simulink library "ForcesHypothese"  (R2018a)
settings: Solver=VariableStepAuto  StartTime=0.0  StopTime=10.0  RelTol=1e-3
values from neighbouring files (symbols this model uses):
  w_alpha = 0    [LimitationVitesse.m]
  w_dist = 0    [LimitationVitesse.m]
settings Model: Creator=thomas.moser  LastModifiedBy=thomas.moser

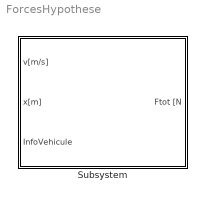
== system ForcesHypothese ==
  Subsystem : Subsystem  mask{rho=1.225, g=9.81}
      mask prompts: rho "Densité de l'air [kg/m^3] :"; g "Accélération gravitationelle [m/s^2] :"

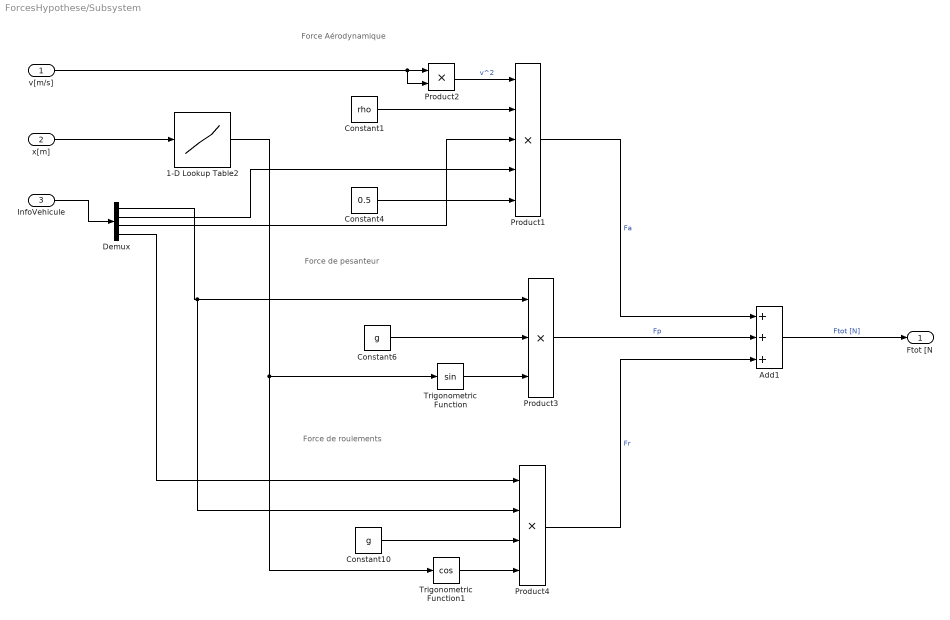
== system ForcesHypothese/Subsystem ==
  note: Force de pesanteur
  note: Force de roulements
  note: Force Aérodynamique
  v[m/s] : Inport
  x[m] : Inport  Port=2
  InfoVehicule : Inport  Port=3
  1-D Lookup Table2 : Lookup_n-D  NumberOfTableDimensions=1  BreakpointsForDimension1=w_dist  Table=w_alpha  InternalRulePriority=Speed  RndMeth=Simplest  InputSameDT=on
  Add1 : Sum  Inputs=+++
  Constant1 : Constant  Value=rho
  Constant10 : Constant  Value=g
  Constant4 : Constant  Value=0.5
  Constant6 : Constant  Value=g
  Demux : Demux
  Product1 : Product  Inputs=5
  Product2 : Product
  Product3 : Product  Inputs=3
  Product4 : Product  Inputs=4
  Trigonometric Function : Trigonometry
  Trigonometric Function1 : Trigonometry  Operator=cos
  Ftot [N : Outport
  wires:
  Constant1/1 -> Product1/2
  1-D Lookup Table2/1 -> Trigonometric Function/1, Trigonometric Function1/1
  v[m/s]/1 -> Product2/2, Product2/1
  Add1/1 -> Ftot [N/1  "Ftot [N]"
  Product4/1 -> Add1/3  "Fr"
  Constant4/1 -> Product1/5
  Constant6/1 -> Product3/2
  x[m]/1 -> 1-D Lookup Table2/1
  Constant10/1 -> Product4/3
  Product3/1 -> Add1/2  "Fp"
  Product2/1 -> Product1/1  "v^2"
  Product1/1 -> Add1/1  "Fa"
  Trigonometric Function1/1 -> Product4/4
  Trigonometric Function/1 -> Product3/3
  InfoVehicule/1 -> Demux/1
  Demux/1 -> Product4/2, Product3/1
  Demux/2 -> Product1/4
  Demux/3 -> Product1/3
  Demux/4 -> Product4/1
